simulink model "Model_2711_re"  (R2024b)
settings: Solver=VariableStepAuto  StartTime=0.0  StopTime=10.0  RelTol=1e-3
values from neighbouring files (symbols this model uses):
  D = [1 0 0 ... (first row only)    [satellite_Magtorq.m]
  Is = diag([0.06, 0.05, 0.06])    [satellite_Magtorq.m]
  Iw = 50e-6    (= 5e-05)    [satellite_Magtorq.m]
  KM = 9.5e-3    (= 0.0095)    [satellite_Magtorq.m]
libraries: aerolibutil x1
settings Model: Creator=LEGION  LastModifiedBy=LEGION

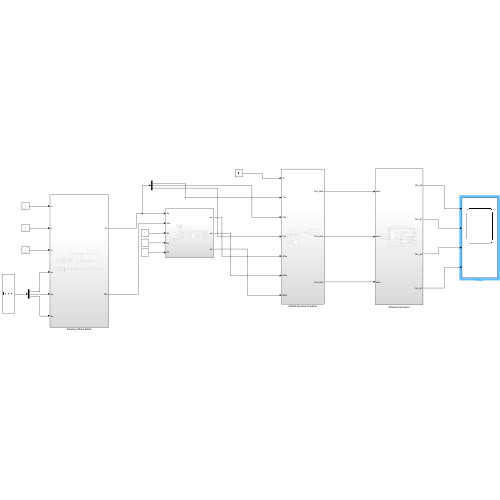
[thumbnail: Simulink's stored preview of the top-level diagram]
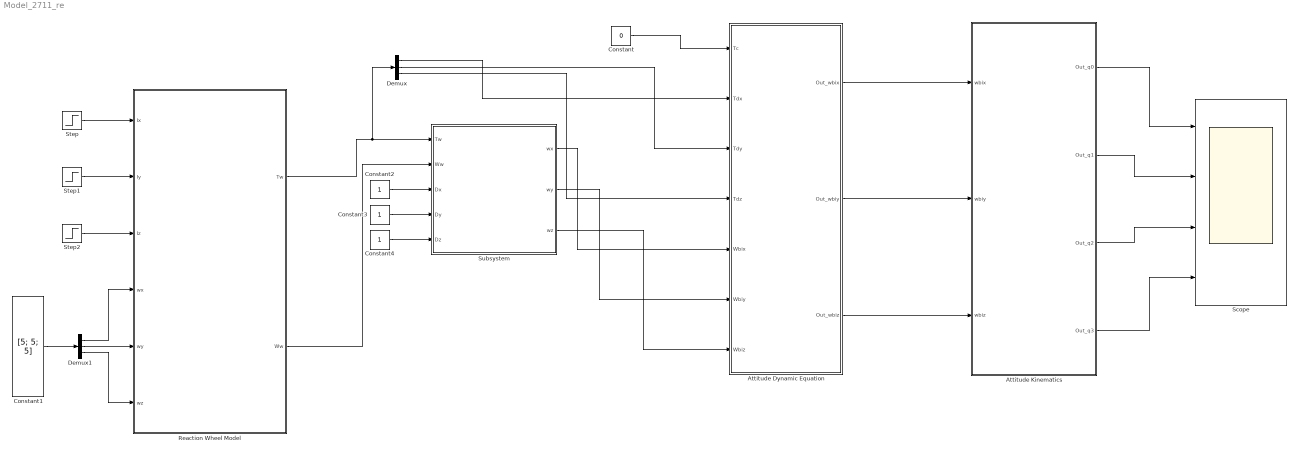
== system Model_2711_re ==
  Attitude Dynamic Equation : Subsystem
  Attitude Kinematics : Subsystem
  Constant : Constant  Value=0
  Constant1 : Constant  Value=[5; 5; 5]
  Constant2 : Constant
  Constant3 : Constant
  Constant4 : Constant
  Demux : Demux  Outputs=3
  Demux1 : Demux  Outputs=3
  Reaction Wheel Model : Subsystem
  Scope : Scope  NumInputPorts=4
  Step : Step  SampleTime=0
  Step1 : Step  SampleTime=0
  Step2 : Step  SampleTime=0
  Subsystem : Subsystem
  wires:
  Reaction Wheel Model/1(Tw) -> Demux/1, Subsystem/1(Tw)
  Reaction Wheel Model/2(Ww) -> Subsystem/2(Ww)
  Subsystem/3(wz) -> Attitude Dynamic Equation/7(Wbiz)
  Subsystem/2(wy) -> Attitude Dynamic Equation/6(Wbiy)
  Subsystem/1(wx) -> Attitude Dynamic Equation/5(Wbix)
  Demux/3 -> Attitude Dynamic Equation/4(Tdz)
  Demux/2 -> Attitude Dynamic Equation/3(Tdy)
  Demux/1 -> Attitude Dynamic Equation/2(Tdx)
  Constant/1 -> Attitude Dynamic Equation/1(Tc)
  Attitude Dynamic Equation/1(Out_wbix) -> Attitude Kinematics/1(wbix)
  Attitude Dynamic Equation/2(Out_wbiy) -> Attitude Kinematics/2(wbiy)
  Attitude Dynamic Equation/3(Out_wbiz) -> Attitude Kinematics/3(wbiz)
  Step/1 -> Reaction Wheel Model/1(Ix)
  Step1/1 -> Reaction Wheel Model/2(Iy)
  Step2/1 -> Reaction Wheel Model/3(Iz)
  Constant1/1 -> Demux1/1
  Demux1/1 -> Reaction Wheel Model/4(wx)
  Demux1/2 -> Reaction Wheel Model/5(wy)
  Demux1/3 -> Reaction Wheel Model/6(wz)
  Attitude Kinematics/1(Out_q0) -> Scope/1
  Attitude Kinematics/2(Out_q1) -> Scope/2
  Attitude Kinematics/3(Out_q2) -> Scope/3
  Attitude Kinematics/4(Out_q3) -> Scope/4
  Constant2/1 -> Subsystem/3(Dx)
  Constant3/1 -> Subsystem/4(Dy)
  Constant4/1 -> Subsystem/5(Dz)

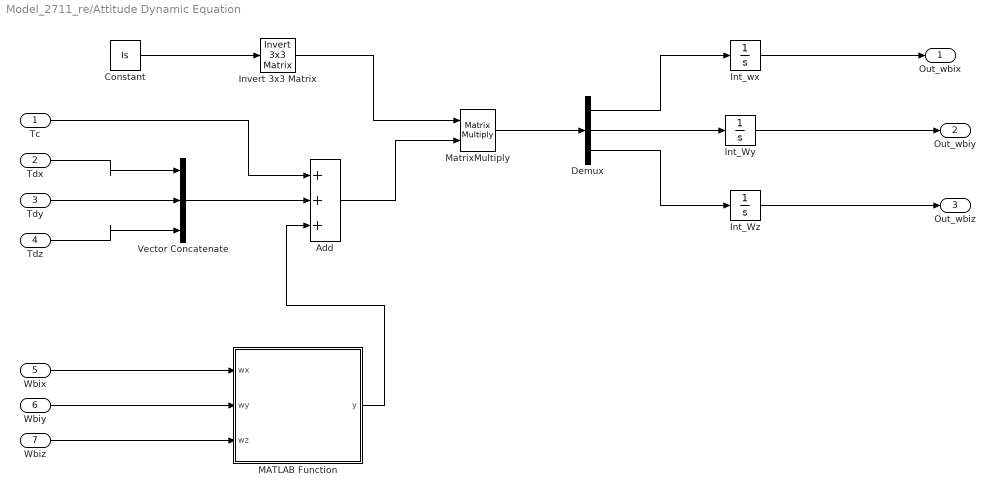
== system Model_2711_re/Attitude Dynamic Equation ==
  Tc : Inport
  Tdx : Inport  Port=2
  Tdy : Inport  Port=3
  Tdz : Inport  Port=4
  Wbix : Inport  Port=5
  Wbiy : Inport  Port=6
  Wbiz : Inport  Port=7
  Add : Sum  Inputs=+++
  Constant : Constant  Value=Is
  Demux : Demux  Outputs=3
  Int_Wy : Integrator
  Int_Wz : Integrator
  Int_wx : Integrator
  Invert 3x3 Matrix : aerolibutil/Invert  3x3 Matrix
  MATLAB Function : MATLAB Function  TreatAsAtomicUnit=on
  MatrixMultiply : Product  Multiplication=Matrix(*)
  Vector Concatenate : Concatenate  NumInputs=3
  Out_wbix : Outport
  Out_wbiy : Outport  Port=2
  Out_wbiz : Outport  Port=3
  wires:
  Demux/1 -> Int_wx/1
  Wbiz/1 -> MATLAB Function/3(wz)
  Int_Wy/1 -> Out_wbiy/1
  MATLAB Function/1(y) -> Add/3
  Add/1 -> MatrixMultiply/2
  Tdz/1 -> Vector Concatenate/3
  Tdx/1 -> Vector Concatenate/1
  Demux/2 -> Int_Wy/1
  Int_wx/1 -> Out_wbix/1
  Demux/3 -> Int_Wz/1
  MatrixMultiply/1 -> Demux/1
  Invert 3x3 Matrix/1 -> MatrixMultiply/1
  Constant/1 -> Invert 3x3 Matrix/1
  Tdy/1 -> Vector Concatenate/2
  Int_Wz/1 -> Out_wbiz/1
  Wbix/1 -> MATLAB Function/1(wx)
  Tc/1 -> Add/1
  Wbiy/1 -> MATLAB Function/2(wy)
  Vector Concatenate/1 -> Add/2

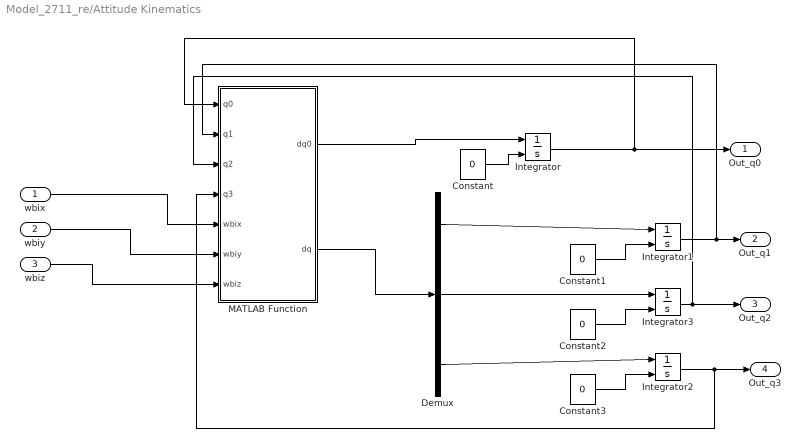
== system Model_2711_re/Attitude Kinematics ==
  wbix : Inport
  wbiy : Inport  Port=2
  wbiz : Inport  Port=3
  Constant{,1..3} (4 alike) : Constant  Value=0
  Demux : Demux  Outputs=3
  Integrator{,1..3} (4 alike) : Integrator  InitialConditionSource=external  InitialCondition=1
  MATLAB Function : MATLAB Function  TreatAsAtomicUnit=on
  Out_q0 : Outport
  Out_q1 : Outport  Port=2
  Out_q2 : Outport  Port=3
  Out_q3 : Outport  Port=4
  wires:
  wbiz/1 -> MATLAB Function/7(wbiz)
  wbiy/1 -> MATLAB Function/6(wbiy)
  wbix/1 -> MATLAB Function/5(wbix)
  MATLAB Function/2(dq) -> Demux/1
  Constant/1 -> Integrator/2
  MATLAB Function/1(dq0) -> Integrator/1
  Demux/1 -> Integrator1/1
  Demux/2 -> Integrator3/1
  Demux/3 -> Integrator2/1
  Constant1/1 -> Integrator1/2
  Constant2/1 -> Integrator3/2
  Constant3/1 -> Integrator2/2
  Integrator/1 -> MATLAB Function/1(q0), Out_q0/1
  Integrator2/1 -> MATLAB Function/4(q3), Out_q3/1
  Integrator3/1 -> MATLAB Function/3(q2), Out_q2/1
  Integrator1/1 -> MATLAB Function/2(q1), Out_q1/1

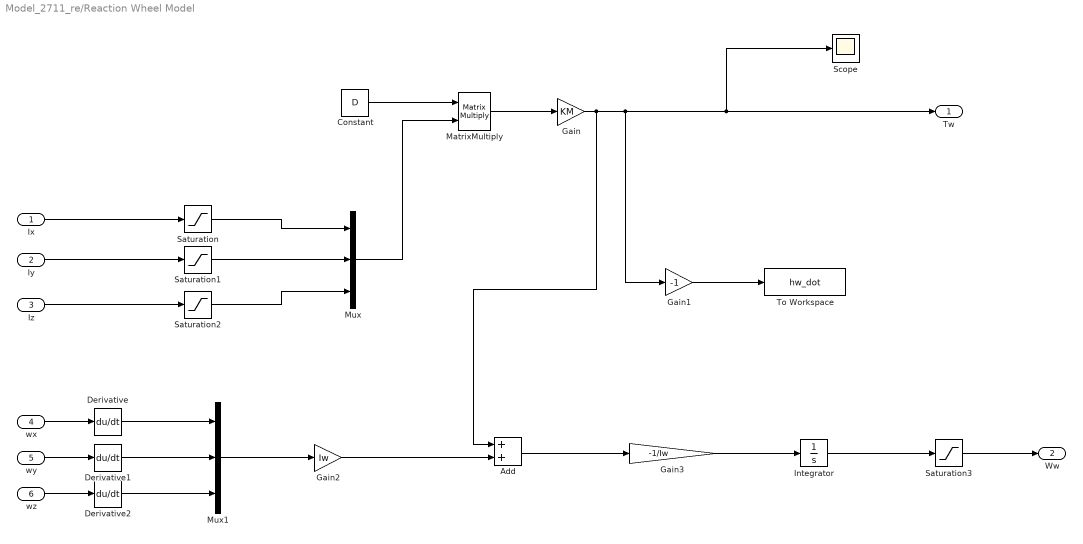
== system Model_2711_re/Reaction Wheel Model ==
  Ix : Inport
  Iy : Inport  Port=2
  Iz : Inport  Port=3
  wx : Inport  Port=4
  wy : Inport  Port=5
  wz : Inport  Port=6
  Add : Sum
  Constant : Constant  Value=D
  Derivative : Derivative
  Derivative1 : Derivative
  Derivative2 : Derivative
  Gain : Gain  Gain=KM
  Gain1 : Gain  Gain=-1
  Gain2 : Gain  Gain=Iw
  Gain3 : Gain  Gain=-1/Iw
  Integrator : Integrator
  MatrixMultiply : Product  Multiplication=Matrix(*)
  Mux : Mux  Inputs=3
  Mux1 : Mux  Inputs=3
  Saturation{,1..3} (4 alike) : Saturate
  Scope : Scope
  To Workspace : ToWorkspace  VariableName=hw_dot  SaveFormat=Timeseries  SampleTime=-1
  Tw : Outport
  Ww : Outport  Port=2
  wires:
  Ix/1 -> Saturation/1
  Iy/1 -> Saturation1/1
  Saturation1/1 -> Mux/2
  Saturation/1 -> Mux/1
  Saturation2/1 -> Mux/3
  Constant/1 -> MatrixMultiply/1
  Mux/1 -> MatrixMultiply/2
  MatrixMultiply/1 -> Gain/1
  Gain/1 -> Add/1, Gain1/1, Scope/1, Tw/1
  Gain1/1 -> To Workspace/1
  Derivative/1 -> Mux1/1
  Derivative1/1 -> Mux1/2
  Derivative2/1 -> Mux1/3
  Mux1/1 -> Gain2/1
  Gain2/1 -> Add/2
  Add/1 -> Gain3/1
  Gain3/1 -> Integrator/1
  Integrator/1 -> Saturation3/1
  Saturation3/1 -> Ww/1
  Iz/1 -> Saturation2/1
  wx/1 -> Derivative/1
  wy/1 -> Derivative1/1
  wz/1 -> Derivative2/1

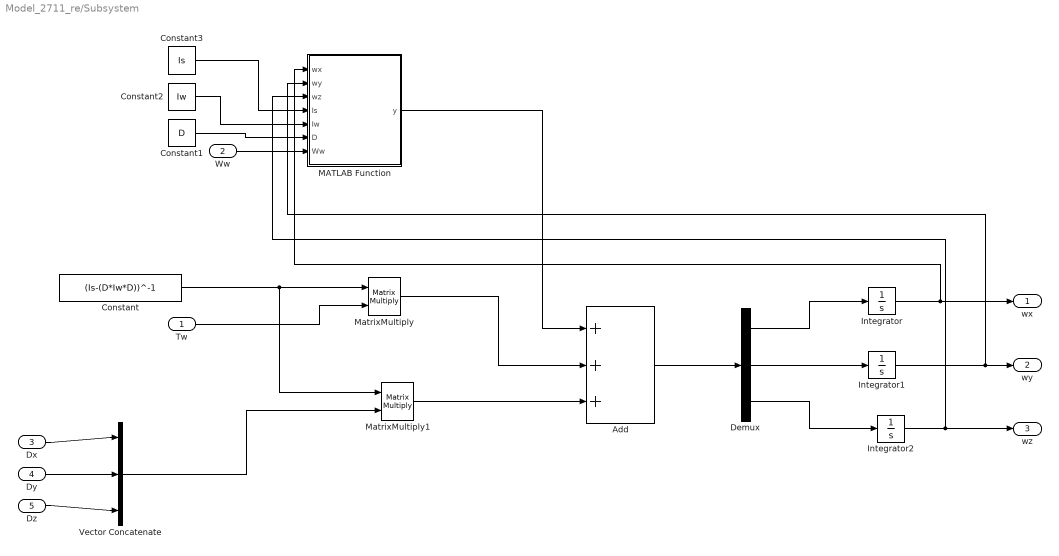
== system Model_2711_re/Subsystem ==
  Tw : Inport
  Ww : Inport  Port=2
  Dx : Inport  Port=3
  Dy : Inport  Port=4
  Dz : Inport  Port=5
  Add : Sum  Inputs=+++
  Constant : Constant  Value=(Is-(D*Iw*D))^-1
  Constant1 : Constant  Value=D
  Constant2 : Constant  Value=Iw
  Constant3 : Constant  Value=Is
  Demux : Demux  Outputs=3
  Integrator : Integrator
  Integrator1 : Integrator
  Integrator2 : Integrator
  MATLAB Function : MATLAB Function  TreatAsAtomicUnit=on
  MatrixMultiply : Product  Multiplication=Matrix(*)
  MatrixMultiply1 : Product  Multiplication=Matrix(*)
  Vector Concatenate : Concatenate  NumInputs=3
  wx : Outport
  wy : Outport  Port=2
  wz : Outport  Port=3
  wires:
  Tw/1 -> MatrixMultiply/2
  Constant/1 -> MatrixMultiply1/1, MatrixMultiply/1
  Dx/1 -> Vector Concatenate/1
  Dy/1 -> Vector Concatenate/2
  Dz/1 -> Vector Concatenate/3
  Vector Concatenate/1 -> MatrixMultiply1/2
  MatrixMultiply1/1 -> Add/3
  MatrixMultiply/1 -> Add/2
  MATLAB Function/1(y) -> Add/1
  Add/1 -> Demux/1
  Demux/3 -> Integrator2/1
  Demux/2 -> Integrator1/1
  Demux/1 -> Integrator/1
  Integrator/1 -> MATLAB Function/1(wx), wx/1
  Integrator1/1 -> MATLAB Function/2(wy), wy/1
  Integrator2/1 -> MATLAB Function/3(wz), wz/1
  Constant1/1 -> MATLAB Function/6(D)
  Ww/1 -> MATLAB Function/7(Ww)
  Constant2/1 -> MATLAB Function/5(Iw)
  Constant3/1 -> MATLAB Function/4(Is)

== matlab function Model_2711_re/Attitude Kinematics/MATLAB Function ==
  data: q0 input; dq0 output; q1 input; q2 input; q3 input; wbix input; wbiy input; wbiz input; dq output
function [dq0, dq] = fcn(q0, q1, q2, q3, wbix, wbiy, wbiz)
    q = [q1; q2; q3];
    skew_symmetric_matrix_qs = [0 -q3 q2;
                               q3 0 -q1;
                              -q2 q1 0];
    dq0 = -0.5 * [wbix; wbiy; wbiz]' * [1];
    dq = 0.5 * ((q0 * eye(3)) + skew_symmetric_matrix_qs) * [wbix; wbiy; wbiz];
end

== matlab function Model_2711_re/Attitude Dynamic Equation/MATLAB Function ==
  data: wx input; y output; wy input; wz input
function y = fcn(wx,wy,wz)
Is =diag([0.06, 0.05, 0.06]);
ww = [0 -wz wy;
     wz 0 -wx;
     -wy wx 0];
y = - inv(Is) * ww * (Is * [wx;wy;wz]);

== matlab function Model_2711_re/Subsystem/MATLAB Function ==
  data: wx input; y output; wy input; wz input; Is input; Iw input; D input; Ww input
function y = fcn(wx,wy,wz,Is,Iw,D,Ww)
ww = [0 -wz wy;
wz 0 -wx;
-wy wx 0];
y = - inv(Is-(D*Iw*D')) * ww * ((Is * [wx;wy;wz]) + (Iw*D*Ww));
